simulink library "vexv5_SD_Logging_Lib"  (R2019b)
settings: Solver=FixedStepAuto  StartTime=0.0  StopTime=10.0  RelTol=1e-3
undefined symbols (not defined in the file): rt_RobotSession
libraries: simulink x1
settings Model: Creator=josea  LastModifiedBy=josea
settings OptimizationCC: EnhancedBackFolding=on  PassReuseOutputArgsAs=Individual arguments  ZeroExternalMemoryAtStartup=off  ZeroInternalMemoryAtStartup=off  MaxStackSize=64  OptimizeBlockOrder=speed  DifferentSizesBufferReuse=on  OptimizationCustomize=off  EfficientTunableParamExpr=on
settings DebuggingCC: ParameterTunabilityLossMsg=error
settings HardwareCC: ProdBitPerPointer=32  ProdBitPerSizeT=32  ProdBitPerPtrDiffT=32  ProdLargestAtomicInteger=Long  ProdLargestAtomicFloat=Double  ProdWordSize=32  ProdHWDeviceType=ARM Compatible->ARM Cortex
settings SFSimCC: MATLABDynamicMemAlloc=off
settings RTWCC: SystemTargetFile=ert.tlc  HardwareBoard=VEX V5 Robot Brain  TLCOptions="-aInlineSetEventsForThisBaseRateFcn=TLC_FALSE -aSuppressMultiTaskScheduler=TLC_FALSE  -aRateBasedStepFcn=0"  TemplateMakefile=ert_default_tmf  GenerateReport=on  Toolchain=GNU Tools for ARM Embedded Processors  IncludeHyperlinkInReport=on  LaunchReport=on  GenerateTraceInfo=on  GenerateTraceReport=on  GenerateTraceReportSl=on  GenerateTraceReportSf=on  GenerateTraceReportEml=on
settings CodeAppCC: ForceParamTrailComments=on  IgnoreCustomStorageClasses=off  OperatorAnnotations=on  SimulinkDataObjDesc=on  SFDataObjDesc=on  InsertBlockDesc=on
settings ERTTargetCC: MatFileLogging=on  ExtModeStaticAllocSize=2048

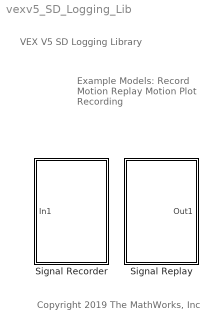
== system vexv5_SD_Logging_Lib ==
  note: Example Models:
      | Record Motion
      | Replay Motion
      | Plot Recording
  note: VEX V5 SD Logging Library
  note: Copyright 2019 The MathWorks, Inc
  Signal Recorder : Subsystem  mask(VEX Signal Recorder){SampleTime=-1}
      mask prompts: SampleTime "Simulink:blkprm_prompts:AllBlksSampleTime"
      mask help:
      | This block is used to save signals into an SD car inserted to the VEX V5 Robot Brain.
      |
      | The block automatically modifies model settings for VEX SD data logging. For more details on manually logging Simulink signals to an SD card see the help for this block.
      |
      | RECORDING TIME: The signals are recorded for corresponding model STOP TIME. If the stop time is set to 'inf' then data is saved to multiple files with time intervals depending on the number of signals logged and the 'sample time'.
      |
      | FILE NAMES: The model name is used to name the log files and session and interval indexes are appended.
      settings: CopyFcn=|
      | set_param(gcs,'HardwareBoard','VEX V5 Robot Brain')
      | set_param(gcs,'MatFileLogging','on')
      mask Help: helpview(fullfile(codertarget.internal.vexv5.getDocRoot,'ug','sd-card-logging.html'))
      mask TypeOptions SampleTime: To Workspace/SampleTime
      mask DialogControl Container2 Prompt: Parameters
      mask DialogControl SampleTime Prompt: Sample time (-1 for inherited):
      mask Display:
      | image(imread('SD_record.PNG'))
      | patch([0.1, 0.1, 0.1, 0.1], [1, 1, 1, 0.1], [1, 1, 1]);
      | color('blue');
      | text(1, 1, 'VEX V5', 'horizontalAlignment', 'right', 'verticalAlignment','top');
  Signal Replay : Subsystem  mask(VEX Signal Replay){sel_session=vexv5_Right_Turn_1__stitched}
      mask prompts: sel_session "RobotSession"
      mask help:
      | This block is used to replay signals recorded using an SD card inserted to the VEX V5 Robot Brain.
      |
      | Signal data is imported to the Simulink model and uploaded to the Robot without the need of re-inserting the SD card in the VEX V5 Robot Brain.
      mask init:
      | mat_name=get_param(gcb,'sel_session');
      | evalin('base',['load(''' mat_name '.mat'');']);
      | Ts=evalin('base','rt_RobotSession.time(2);');
      mask Help: For more help using this block please contact roboticsarena@mathworks.com
      mask DialogControl Container2 Prompt: Set Data
      mask DialogControl Control2 Prompt: Import Session
      mask DialogControl Control2 Callback:
      | mat_file=vexImportSession;
      | if ~isempty(mat_file)
      | set_param(gcb,'sel_session',mat_file);
      | end
      mask Display:
      | image(imread('SD_play.PNG'))
      | patch([0.1, 0.1, 0.1, 0.1], [1, 1, 1, 0.1], [1, 1, 1]);
      | color('blue');
      | text(1, 1, 'VEX V5', 'horizontalAlignment', 'right', 'verticalAlignment','top');

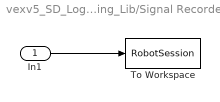
== system vexv5_SD_Logging_Lib/Signal Recorder ==
  In1 : Inport
  To Workspace : ToWorkspace  VariableName=RobotSession  SaveFormat=Structure With Time  SampleTime=SampleTime
  wires:
  In1/1 -> To Workspace/1

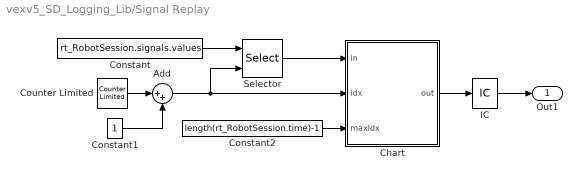
== system vexv5_SD_Logging_Lib/Signal Replay ==
  Add : Sum  Inputs=|++
  Chart : Stateflow chart  TreatAsAtomicUnit=on
  Constant : Constant  Value=rt_RobotSession.signals.values
  Constant1 : Constant
  Constant2 : Constant  Value=length(rt_RobotSession.time)-1
  Counter Limited : simulink/Sources/Counter Limited  uplimit=length(rt_RobotSession.time)-1  tsamp=Ts
  IC : InitialCondition  Value=0
  Selector : Selector  NumberOfDimensions=2  InputPortWidth=length(rt_RobotSession.time)  IndexOptions=Index vector (port),Index vector (dialog)  Indices=[1 3],1:rt_RobotSession.signals.dimensions  OutputSizes=1,1
  Out1 : Outport
  wires:
  IC/1 -> Out1/1
  Constant2/1 -> Chart/3(maxIdx)
  Chart/1(out) -> IC/1
  Selector/1 -> Chart/1(in)
  Constant1/1 -> Add/2
  Add/1 -> Chart/2(idx), Selector/2
  Counter Limited/1 -> Add/1
  Constant/1 -> Selector/1

== stateflow chart vexv5_SD_Logging_Lib/Signal Replay/Chart ==
  state Increment
    out=in;
  state Hold
  (default) -> Increment
  Increment -> Hold : [idx>maxIdx]
  data: in input; out output; idx input; maxIdx input
